simulink model "KTB1_SMAH"  (R2020a)
settings: Solver=ode45  StartTime=0.0  StopTime=120  RelTol=1e-3
values from neighbouring files (symbols this model uses):
  max_X = 5100    [SAP.m]
  max_XX = 2    [SAP.m]
  max_XXX = 0.05    [SAP.m]
  max_XXXX = 1050    [SAP.m]
  max_XXXXX = 15    [SAP.m]
  min_X = 0    [SAP.m]
  min_XX = 0    [SAP.m]
  min_XXX = 0    [SAP.m]
  min_XXXX = 0    [SAP.m]
  min_XXXXX = 0    [SAP.m]
  noiseseed = use2ndFcn    (= 1)    [SAP.m]
  noiseseed_X = use2ndFcn_X    (= 1)    [SAP.m]
  noiseseed_XX = use2ndFcn_XX    (= 1)    [SAP.m]
  noiseseed_XXX = use2ndFcn_XXX    (= 1)    [SAP.m]
  noiseseed_XXXX = use2ndFcn_XXXX    (= 1)    [SAP.m]
  noiseseed_XXXXX = use2ndFcn_XXXXX    (= 1)    [SAP.m]
  std = 0.025    [SAP.m]
  std_X = 0.025    [SAP.m]
  std_XX = 0.025    [SAP.m]
  std_XXX = 0.025    [SAP.m]
  std_XXXX = 0.025    [SAP.m]
  std_XXXXX = 0.025    [SAP.m]
  T_2 = T90_2/(24*60)/3.89    (= 0.000892602113682)    [SAP.m]
  T_8 = T90_8/(24*60)/11.7724    (= 0.00117978397683)    [SAP.m]
  T_X_2 = T90_X_2/(24*60)/3.89    (= 0.000892602113682)    [SAP.m]
  T_X_8 = T90_X_8/(24*60)/11.7724    (= 0.00117978397683)    [SAP.m]
  T_XX_2 = T90_XX_2/(24*60)/3.89    (= 0.000892602113682)    [SAP.m]
  T_XX_8 = T90_XX_8/(24*60)/11.7724    (= 0.00117978397683)    [SAP.m]
  T_XXX_2 = T90_XXX_2/(24*60)/3.89    (= 0.000892602113682)    [SAP.m]
  T_XXXX_2 = T90_XXXX_2/(24*60)/3.89    (= 0.000892602113682)    [SAP.m]
  T_XXXXX_2 = T90_XXXXX_2/(24*60)/3.89    (= 0.000892602113682)    [SAP.m]
  use2ndFcn = 1    [SAP.m]
  use2ndFcn_X = 1    [SAP.m]
  use2ndFcn_XX = 1    [SAP.m]
  use2ndFcn_XXX = 1    [SAP.m]
  use2ndFcn_XXXX = 1    [SAP.m]
  use2ndFcn_XXXXX = 1    [SAP.m]
  useideal = 1    [SAP.m]
  useideal_X = 1    [SAP.m]
  useideal_XX = 1    [SAP.m]
  useideal_XXX = 1    [SAP.m]
  useideal_XXXX = 1    [SAP.m]
  useideal_XXXXX = 1    [SAP.m]
  useidealac = 1    [SAP.m]
  useidealac_X = 1    [SAP.m]
  useidealac_XX = 1    [SAP.m]
  useidealac_XXX = 1    [SAP.m]
  useidealac_XXXX = 1    [SAP.m]
  useidealac_XXXXX = 1    [SAP.m]
  usenoise = 0    [SAP.m]
  usenoise_X = 0    [SAP.m]
  usenoise_XX = 0    [SAP.m]
  usenoise_XXX = 0    [SAP.m]
  usenoise_XXXX = 0    [SAP.m]
  usenoise_XXXXX = 0    [SAP.m]
libraries: simulink x6
(part 2 of 2)

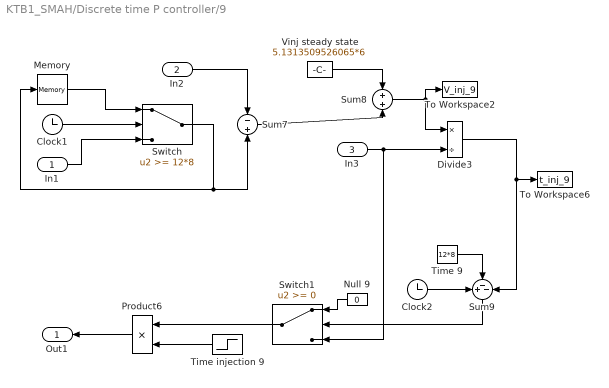
== system KTB1_SMAH/Discrete time P controller/9 ==
  In1 : Inport
  In2 : Inport  Port=2
  In3 : Inport  Port=3
  Clock1 : Clock
  Clock2 : Clock
  Divide3 : Product  Inputs=*/
  Memory : Memory
  Null 9 : Constant  Value=0
  Product6 : Product
  Sum7 : Sum  Inputs=-+
  Sum8 : Sum
  Sum9 : Sum  Inputs=+--
  Switch : Switch  Threshold=12*8
  Switch1 : Switch
  Time 9 : Constant  Value=12*8
  Time injection 9 : Step  Time=12*8  SampleTime=0
  To Workspace2 : ToWorkspace  VariableName=V_inj_9  SaveFormat=Timeseries  SampleTime=-1
  To Workspace6 : ToWorkspace  VariableName=t_inj_9  SaveFormat=Timeseries  SampleTime=-1
  Vinj steady state : Constant  Value=5.1313509526065*6
  Out1 : Outport  VectorParamsAs1DForOutWhenUnconnected=off
  wires:
  In1/1 -> Switch/3
  Time injection 9/1 -> Product6/2
  Switch/1 -> Memory/1, Sum7/2
  Time 9/1 -> Sum9/2
  Switch1/1 -> Product6/1
  Clock1/1 -> Switch/2
  Memory/1 -> Switch/1
  Null 9/1 -> Switch1/1
  Divide3/1 -> Sum9/3, To Workspace6/1
  Clock2/1 -> Sum9/1
  In2/1 -> Sum7/1
  Vinj steady state/1 -> Sum8/1
  In3/1 -> Switch1/3, Divide3/2
  Sum9/1 -> Switch1/2
  Sum7/1 -> Sum8/2
  Product6/1 -> Out1/1
  Sum8/1 -> Divide3/1, To Workspace2/1

== matlab function KTB1_SMAH/M-101 ==
  data: y output; u input
function y  = MX(u) 

% inputs
Q_R = u(1);
Q_M = u(2);
C_LAC_M = u(3);
C_N_M = u(4);
C_X_S = u(5);
C_LAC_S = u(6);
C_N_S = u(7);
C_MEV_S = u(8);

%C_LAC_M=10;
%C_N_M=2;

beta=1.9;

%remember C_LAC_R=C_LAC_S C_N_R=C_N_S

y=zeros(5,1);
y(1) = C_X_S*beta*Q_R/(Q_M+Q_R); %C_X_F
y(2) = (C_LAC_M*Q_M+C_LAC_S*Q_R)/(Q_M+Q_R); %C_LAC_F
y(3) = (C_N_M*Q_M+C_N_S*Q_R)/(Q_M+Q_R); %C_N_F
y(4) = C_MEV_S*Q_R/(Q_M+Q_R); %C_MEV_F
y(5) = (Q_M+Q_R); % Q_F

== matlab function KTB1_SMAH/C-101 ==
  data: u input size=6; y output
 function y  = CF1(u)
% X=0.99; %separation factor
%Q4=QP1; volumetric capacity of the centrifuge

%inputs
C_X_T = u(1);
C_LAC_T = u(2);
C_N_T = u(3);
C_MEV_T = u(4);
Q_T = u(5);
X = u(6);

y=zeros(5,1);

y(1)=(1-X)*C_X_T;
y(2)=C_LAC_T;
y(3)=C_N_T;
y(4)=C_MEV_T;
y(5)= Q_T;

== matlab function KTB1_SMAH/Purge ==
  data: u input size=7; y output
function y = PU(u)

% inputs
C_X_S = u(1);
C_LAC_S = u(2);
C_N_S = u(3);
C_MEV_S = u(4);
Q_M=u(5);
Q_C=u(6);
Q_P=u(7);

%F_purge=0.13;
%R=0.8;
% Q1=1.6; %l/h
%QC=1.8;
% F_purge*Q_C
%Q_P=Q_C-0.8*Q_1;

y=zeros(2,1);
y(1) = (Q_C-Q_P)/Q_M; % RR
y(2) = (Q_C-Q_P); % Q_R

== matlab function KTB1_SMAH/C-102 ==
  data: u input size=6; y output
 function y  = CF2(u)
% X=0.99; %separation factor
%Q4=QP1; volumetric capacity of the centrifuge

%inputs
X = u(1); %separation factor
C_X_T = u(2);
C_LAC_T = u(3);
C_N_T = u(4);
C_MEV_T = u(5);
Q_T = u(6);


y=zeros(5,1);

y(1)=(1-X)*C_X_T;
y(2)=C_LAC_T;
y(3)=C_N_T;
y(4)=C_MEV_T;
y(5)= Q_T;

== matlab function KTB1_SMAH/VSP-101 ==
  data: u input size=2; y output size=2
function y  = VSP(u)

%input
%time=u(1);
Q=u(1);
n=u(2);

dim=2;

y=zeros(dim,1);

% output

y(1)=Q;
y(2)=(-0.085*Q^2 - 0.0000329*Q*n + 0.0000155555555555556*n^2)/10.2024665317458;

% -0.085x^(2)-0.0000329*2900x+0.0000155555555555556*2900

%10.199773339984

end

== matlab function KTB1_SMAH/NF-101 ==
  data: u input size=5; y output size=9
function y  = NF(u)
%% parameters for nanofiltration 
% a DOW NF90 nanofiltration membrane has been chosen. This type of membrane
% has been used in pharmaceutical applications for API filtrations (title
% reference: Removal of antibiotics from a model wastewater by RO/NF membranes)
%A=0.398443840087261; %membrane surface area [m^2] 
A=0.3984033;
Jw=57.90; %permeate flowrate at 8 bar pressure [l/m^2/h]
Res=Jw/8; %[l/m^2/h/bar]
% [LAC N MEV-H]


%input
C_LAC_4=u(1);
C_N_4=u(2);
C_MEV_4=u(3);
Q_IN=u(4);
P=u(5);


tlim=1; %h
dim=9;

y=zeros(dim,1);

%rejection factors based on molecular weights of similar compounds
if P<=8
    Rej=[0.9; 0.79; 0.00002*P^4 - 0.0018*P^3 + 0.0145*P^2 + 0.0849*P + 0.22248];
else
    Rej=[0.9; 0.79; 0.00002*8^4 - 0.0018*8^3 + 0.0145*8^2 + 0.0849*8 + 0.22248];
end
%Rej=[0.9; 0.79; 0.99];
% y=zeros(4,1);
% tlim=500;

%% output
%y=[Q_P2,Q_R,C_LAC_R,C_N_R,C_MEV_R,C_LAC_P2,C_N_P2,C_MEV_P2]
% if time>=0 && time<tlim
    y(1)=A*Res*P;%permeate volumetric flowrate [l/h];(ref: Continuous purification of
    %active pharmaceutical ingredients using multistage organic solvent nanofiltration membrane cascade)
    y(2)=Q_IN-y(1); %balance on centrifugation+filtration
    y(3)=(Q_IN*C_LAC_4)/(y(2)+y(1)*(1-Rej(1)));%species balance--retentate stream
    y(4)=(Q_IN*C_N_4)/(y(2)+y(1)*(1-Rej(2)));%species balance--retentate stream
    y(5)=(Q_IN*C_MEV_4)/(y(2)+y(1)*(1-Rej(3)));%species balance--retentate stream
    y(6)=y(3)*(1-Rej(1));%LAC
    y(7)=y(4)*(1-Rej(2));%N
    y(8)=y(5)*(1-Rej(3));%MEV
    y(9)=Rej(3);
%else
%    for i=1:dim
%        y(i)=0;
%    end
%end
end

== matlab function KTB1_SMAH/HC-101 ==
  data: u input; y output
function y  = HC(u)

%inputs
Q_S=u(1);
Q_C=u(2);
C_X_S=u(3);
C_LAC_S=u(4);
C_N_S=u(5);
C_MEV_S=u(6);
% Q_R=u(7); % Serve soltanto per Fpurge, eliminabile

%parameters
%R=0.8;
beta=1.6;
%F_purge=0.13;

y=zeros(5,1);

y(1) = (C_X_S*Q_S-beta*C_X_S*Q_C)/(Q_S-Q_C); % C_X
y(2) = C_LAC_S;
y(3) = C_N_S;
y(4) = C_MEV_S;
%y(5) = 1-Q_R/Q_C;
y(5) = Q_S-Q_C;

== matlab function KTB1_SMAH/Controller settings ==
  data: u input size=1; y output size=4
function y  = CN(u)

%inputs
err=u(1);

y=zeros(4,1);
y(1) = -2411.68044009728/310 -30*err; % P
y(2) = y(1)/599.84*1.7; % I
y(3) = -721.322122263916; % D
y(4) = 0.41482994666475; % N
